simulink model "colas_lv_nonlin"  (Simulink 2.09)
settings: Solver=ode45  StartTime=0.0  StopTime=100  MaxStep=1  RelTol=1e-5  AbsTol=1e-5
settings Model: SaveTime=off  SaveOutput=off  ConsistencyChecking=off  RTWTemplateMakefile=grt_unix.tmf

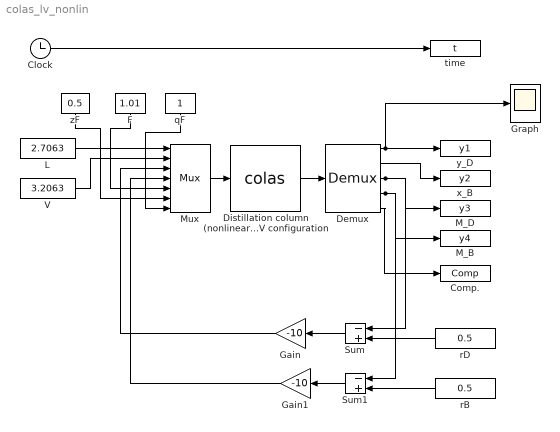
== system colas_lv_nonlin ==
  Clock : Clock
  Comp. : ToWorkspace  VariableName=Comp  SampleTime=0
      settings: Buffer=1000
  Demux : Demux  Outputs=[1,1,1,1,41]
  Distillation column (nonlinear)  LV configuration : S-Function  FunctionName=colas
  F : Constant  Orientation=down  Value=1.01
  Gain : Gain  Orientation=left  Gain=-10
  Gain1 : Gain  Orientation=left  Gain=-10
  Graph : Scope
      settings: TickLabels=on  TimeRange=50  YMin=0.98  YMax=1  SaveToWorkspace=off  SaveName=ScopeData
  L : Constant  Value=2.7063
  M_B : ToWorkspace  VariableName=y4  SampleTime=0
      settings: Buffer=1000
  M_D : ToWorkspace  VariableName=y3  SampleTime=0
      settings: Buffer=1000
  Mux : Mux  Inputs=7
  Sum : Sum  Orientation=left  Inputs=-+
  Sum1 : Sum  Orientation=left  Inputs=-+
  V : Constant  Value=3.2063
  qF : Constant  Orientation=down  Value=1
  rB : Constant  Orientation=left  Value=0.5
  rD : Constant  Orientation=left  Value=0.5
  time : ToWorkspace  VariableName=t  SampleTime=0
      settings: Buffer=1000
  x_B : ToWorkspace  VariableName=y2  SampleTime=0
      settings: Buffer=1000
  y_D : ToWorkspace  VariableName=y1  SampleTime=0
      settings: Buffer=1000
  zF : Constant  Orientation=down  Value=0.5
  wires:
  qF/1 -> Mux/7
  Demux/1 -> Graph/1, y_D/1
  Gain1/1 -> Mux/4
  Sum1/1 -> Gain1/1
  rB/1 -> Sum1/2
  Demux/4 -> Sum1/1, M_B/1
  Demux/3 -> Sum/1, M_D/1
  Gain/1 -> Mux/3
  rD/1 -> Sum/2
  Sum/1 -> Gain/1
  Mux/1 -> Distillation column (nonlinear)  LV configuration/1
  Demux/2 -> x_B/1
  Distillation column (nonlinear)  LV configuration/1 -> Demux/1
  Clock/1 -> time/1
  zF/1 -> Mux/6
  V/1 -> Mux/2
  F/1 -> Mux/5
  Demux/5 -> Comp./1
  L/1 -> Mux/1
